simulink model "FBL_sim"  (R2024b)
settings: Solver=VariableStepAuto  StartTime=0.0  StopTime=15  FixedStep=1e-5  MaxStep=0.001  RelTol=1e-3
values from neighbouring files (symbols this model uses):
  Ampdes = 2.2    [Chapter2.m]    (also in FBL.m; LinearControl.m; SlidingMode.m; control.m)
  Biasdes = 3.3    [Chapter2.m]    (also in FBL.m; LinearControl.m; SlidingMode.m; control.m)
  Freqdes = 2*pi/6    (= 1.0471975512)    [Chapter2.m]    (also in FBL.m; LinearControl.m; SlidingMode.m; control.m)
  Phasedes = 3*pi/2    (= 4.71238898038)    [Chapter2.m]    (also in FBL.m; LinearControl.m; SlidingMode.m; control.m)
  x_0 = [1; 7; 7]    [Chapter2.m]    (also in FBL.m; LinearControl.m; SlidingMode.m; control.m)
libraries: slpidlib x1
settings Model: Creator=Roberto  LastModifiedBy=robyr
settings RTWCC: GPUComputeCapability=3.5

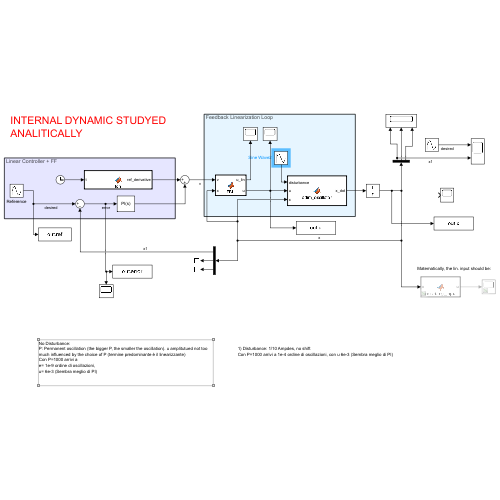
[thumbnail: Simulink's stored preview of the top-level diagram]
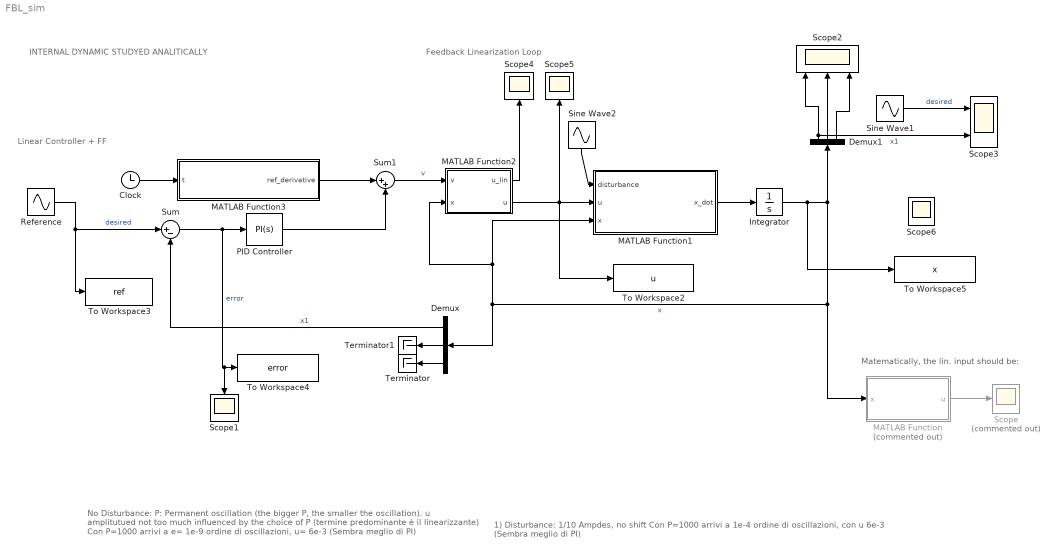
== system FBL_sim ==
  note: No Disturbance:
      | P: Permanent oscillation (the bigger P, the smaller the oscillation). u amplitutued not too much influenced by the choice of P (termine predominante è il linearizzante)
      | Con P=1000 arrivi a
      | e= 1e-9 ordine di oscillazioni,
      | u= 6e-3 (Sembra meglio di PI)
  note: INTERNAL DYNAMIC STUDYED ANALITICALLY
  note: Matematically, the lin. input should be:
  note: Linear Controller + FF
  note: Feedback Linearization Loop
  note: 1) Disturbance: 1/10 Ampdes, no shift
      | Con P=1000 arrivi a 1e-4 ordine di oscillazioni, con u 6e-3 (Sembra meglio di PI)
  Clock : Clock
  Demux : Demux  Outputs=3
  Demux1 : Demux  Outputs=3
  Integrator : Integrator  InitialCondition=x_0
  MATLAB Function : MATLAB Function  Commented=on  TreatAsAtomicUnit=on
  MATLAB Function1 : MATLAB Function  TreatAsAtomicUnit=on
  MATLAB Function2 : MATLAB Function  TreatAsAtomicUnit=on
  MATLAB Function3 : MATLAB Function  TreatAsAtomicUnit=on
  PID Controller : slpidlib/PID Controller  Controller=PI  Form=Parallel  TimeDomain=Continuous-time  UseExternalTs=off  SampleTime=-1  IntegratorMethod=Forward Euler  FilterMethod=Forward Euler  ControllerParametersSource=internal  P=10  I=2  UseKiTs=off  D=5  UseExternalDerivativeSource=off  N=100  UseFilter=on  TunerSelectOption=Transfer Function Based (PID Tuner App)  InitialConditionSource=internal  InitialConditionForIntegrator=0  InitialConditionForFilter=0  DifferentiatorICPrevScaledInput=0  ExternalReset=none  TrackingMode=off  Kt=1  LimitOutput=off  SatLimitsSource=internal  UpperSaturationLimit=inf  LowerSaturationLimit=-inf  LinearizeAsGain=on  AntiWindupMode=none  Kb=1  LimitIntegrator=off  UpperIntegratorSaturationLimit=inf  LowerIntegratorSaturationLimit=-inf  POutMin=[]  POutMax=[]  IOutMin=[]  IOutMax=[]  DOutMin=[]  DOutMax=[]  NOutMin=[]  NOutMax=[]  SumOutMin=[]  SumOutMax=[]  SaturationOutMin=[]  SaturationOutMax=[]  PParamMin=[]  PParamMax=[]  IParamMin=[]  IParamMax=[]  DParamMin=[]  DParamMax=[]  NParamMin=[]  NParamMax=[]  KbParamMin=[]  KbParamMax=[]  KtParamMin=[]  KtParamMax=[]  KbOutMin=[]  KbOutMax=[]  KtOutMin=[]  KtOutMax=[]  IntegratorOutMin=[]  IntegratorOutMax=[]  FilterOutMin=[]  FilterOutMax=[]  SumI1OutMin=[]  SumI1OutMax=[]  SumI2OutMin=[]  SumI2OutMax=[]  SumI3OutMin=[]  SumI3OutMax=[]  SumI4OutMin=[]  SumI4OutMax=[]  SumDOutMin=[]  SumDOutMax=[]  DifferentiatorOutMin=[]  DifferentiatorOutMax=[]  FilterDiffOutCoefMin=[]  FilterDiffOutCoefMax=[]  ReciprocalOutMin=[]  ReciprocalOutMax=[]  SumDenOutMin=[]  SumDenOutMax=[]  SumNumOutMin=[]  SumNumOutMax=[]  DivideOutMin=[]  DivideOutMax=[]  UdiffTsProdOutMin=[]  UdiffTsProdOutMax=[]  NTsProdOutMin=[]  NTsProdOutMax=[]  UintegralTsProdOutMin=[]  UintegralTsProdOutMax=[]  UngainTsProdOutMin=[]  UngainTsProdOutMax=[]  ClampingZeroOutDataTypeStr=Inherit: Inherit via back propagation  ClampingZeroOutMin=[]  ClampingZeroOutMax=[]  FilterDenConstantOutDataTypeStr=Inherit: Inherit via back propagation  FilterDenConstantOutMin=[]  FilterDenConstantOutMax=[]  PCopyOutDataTypeStr=Inherit: Inherit via back propagation  PCopyOutMin=[]  PCopyOutMax=[]  NCopyOutDataTypeStr=Inherit: Inherit via back propagation  NCopyOutMin=[]  NCopyOutMax=[]  IntegratorContinuousStateAttributes=''  IntegratorStateMustResolveToSignalObject=off  IntegratorRTWStateStorageClass=Auto  FilterContinuousStateAttributes=''  FilterStateMustResolveToSignalObject=off  FilterRTWStateStorageClass=Auto  ParallelPVariant=InternalParameters  IdealPVariant=Disabled  IVariant=InternalParameters  DVariant=Disabled  IntegratorVariant=Continuous  SatVariant=Disabled  AWVariant=Passthrough  PCopyVariant=Disabled  TRVariant=Disabled  FdbkBlocksVariant=Forward  IdealPFdbkVariant=Disabled  SatFdbkVariant=Disabled  DerivativeFilterVariant=Disabled  NVariant=Disabled  NCopyVariant=Disabled_SignalSpec  FilterICVariant=Disabled  IntegratorICVariant=InternalICs  ExternalResetVariant=Disabled  TRSumVariant=Passthrough  SumFdbkVariant=Disabled  SumVariant=Sum_PI  TsampFilterVariant=InternalTs  TsampNgainVariant=Passthrough  TsampIntegralVariant=Disabled_SignalSpec  ExternalSaturationOutDataTypeStr=Inherit: Same as second input  DerivativeSourceVariant=Disabled  PreIntVariant=InternalPreInt
  Reference : Sin  Amplitude=Ampdes  Bias=Biasdes  Frequency=Freqdes  Phase=Phasedes  SampleTime=0
  Scope : Scope  Commented=on
  Scope{1,4..6} (4 alike) : Scope
  Scope2 : Scope  NumInputPorts=3
  Scope3 : Scope  NumInputPorts=2
  Sine Wave1 : Sin  Amplitude=Ampdes  Bias=Biasdes  Frequency=Freqdes  Phase=Phasedes  SampleTime=0
  Sine Wave2 : Sin  Amplitude=Ampdes/10  Frequency=Freqdes*100  Phase=Phasedes  SampleTime=0
  Sum : Sum  Inputs=|+-
  Sum1 : Sum  Inputs=|++
  Terminator : Terminator
  Terminator1 : Terminator
  To Workspace2 : ToWorkspace  VariableName=u  SaveFormat=Timeseries  SampleTime=-1
  To Workspace3 : ToWorkspace  VariableName=ref  SaveFormat=Timeseries  SampleTime=-1
  To Workspace4 : ToWorkspace  VariableName=error  SaveFormat=Timeseries  SampleTime=-1
  To Workspace5 : ToWorkspace  VariableName=x  SaveFormat=Timeseries  SampleTime=-1
  wires:
  MATLAB Function1/1(x_dot) -> Integrator/1
  Demux1/2 -> Scope2/2
  Demux/1 -> Sum/2  "x1"
  Demux/3 -> Terminator/1
  Demux1/3 -> Scope2/3
  Reference/1 -> To Workspace3/1, Sum/1  "desired"
  Sum/1 -> Scope1/1, To Workspace4/1, PID Controller/1  "error"
  Integrator/1 -> To Workspace5/1, MATLAB Function2/2(x), MATLAB Function1/3(x), Demux/1, MATLAB Function/1(x), Demux1/1  "x"
  Demux/2 -> Terminator1/1
  MATLAB Function2/2(u) -> Scope5/1, To Workspace2/1, MATLAB Function1/2(u)
  MATLAB Function2/1(u_lin) -> Scope4/1
  MATLAB Function/1(u) -> Scope/1
  Sum1/1 -> MATLAB Function2/1(v)  "v"
  PID Controller/1 -> Sum1/2
  Sine Wave1/1 -> Scope3/1  "desired"
  Demux1/1 -> Scope2/1, Scope3/2  "x1"
  Clock/1 -> MATLAB Function3/1(t)
  MATLAB Function3/1(ref_derivative) -> Sum1/1
  Sine Wave2/1 -> MATLAB Function1/1(disturbance)

== matlab function FBL_sim/MATLAB Function1 ==
  data: disturbance input; u input; x_dot output; x input
function x_dot = adim_oscillator(disturbance, u, x)
n=9;
b=0.1;
a=b^-3;
x_dot = [-x(1)+a/(1+x(3)^n) + a*u + disturbance;...
        -x(2)+x(1);...
        -x(3)+ x(2);];

== matlab function FBL_sim/MATLAB Function2 ==
  data: u_lin output; v input; u output; x input
function [u_lin, u] = FBL(v, x)
n=9;
b=0.1;
a=b^-3;

%Identifie f,g,h:

fx = [-x(1)+a/(1+x(3)^n);...
        -x(2)+x(1);...
        -x(3)+ x(2);];

gx = [a; 0; 0];
%hx=x(1);

grad_h=[1, 0, 0];
lie_1= lie_derivative(grad_h, gx); %Thats =/0, so r=1 (2 Hidden dyn)
u= 1/lie_1 * (-lie_derivative(grad_h,fx) + v);

%Debug: is the linearizing input what we expect?
u_lin= 1/lie_1 * (-lie_derivative(grad_h,fx));

%La Lie Derivative è un operatore che data una riga grad( è un gradiente) 
% e una colonna fx, calcola il prodotto scalare tra essi.
function lie=lie_derivative(grad, fx)
lie= grad * fx;

== matlab function FBL_sim/MATLAB Function ==
  data: x input; u output
function u = linearizing_input(x)
n=9;
b=0.1;
a=b^-3;
u= -1/a*(-x(1)+a/(1+x(3)^n));

== matlab function FBL_sim/MATLAB Function3 ==
  data: t input; ref_derivative output
function ref_derivative = fcn(t)

Ampdes=2.2 ;
Freqdes= 2*pi/6; 
Phasedes= 3*pi/2;


ref_derivative = Ampdes * Freqdes * cos(Freqdes * t + Phasedes);
